simulink model "RRR_arm"  (R2017a)
settings: Solver=FixedStepAuto  StartTime=0.0  StopTime=15  FixedStep=0.1  RelTol=1e-3  EnableMultiTasking=on
settings Model: Creator=PaiChihYun  LastModifiedBy=tonypai
settings OptimizationCC: LifeSpan=inf
settings DebuggingCC: SFUnexpectedBacktrackingDiag=warning  SFNoUnconditionalDefaultTransitionDiag=warning  SFExecutionAtInitializationDiag=none
settings GRTTargetCC: TargetLangStandard=C89/C90 (ANSI)  GeneratePreprocessorConditionals=Disable all
settings ConfigComp: CovMetricSettings=dw  CovHtmlReporting=on  CovSaveCumulativeToWorkspaceVar=on  CovSaveSingleToWorkspaceVar=on  CovExternalEMLEnable=off

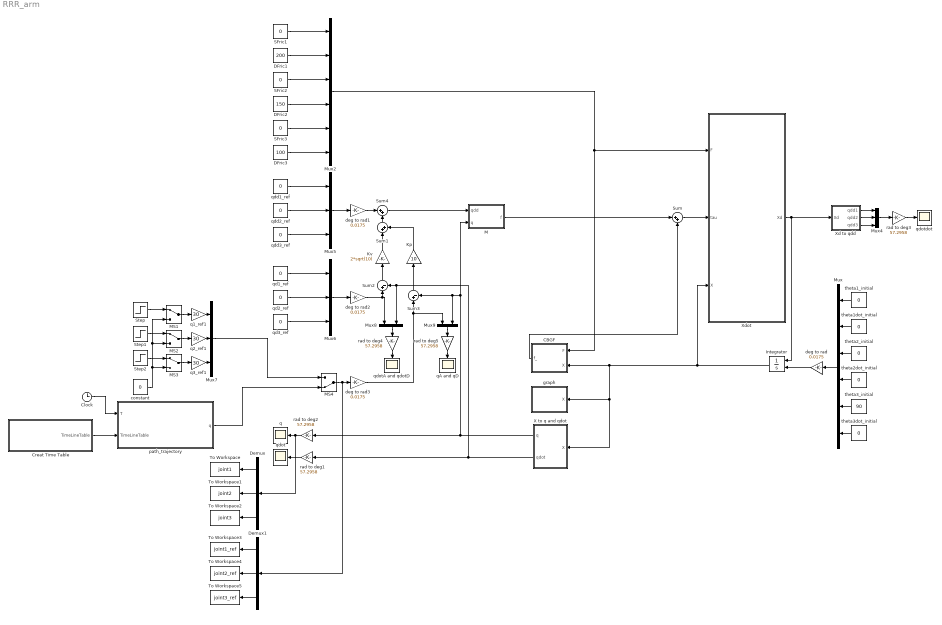
== system RRR_arm ==
  CBGF : MATLAB Function  TreatAsAtomicUnit=on
  Clock : Clock
  Creat Time Table : MATLAB Function  TreatAsAtomicUnit=on
  DFric1 : Constant  Value=200
  DFric2 : Constant  Value=150
  DFric3 : Constant  Value=100
  Demux : Demux  Outputs=3
  Demux1 : Demux  Outputs=3
  Integrator : Integrator  InitialConditionSource=external
  Kp : Gain  Gain=10
  Kv : Gain  Gain=2*sqrt(10)
  M : MATLAB Function  TreatAsAtomicUnit=on
  MS1 : ManualSwitch
  MS2 : ManualSwitch
  MS3 : ManualSwitch
  MS4 : ManualSwitch  CurrentSetting=0
  Mux : Mux  Inputs=6
  Mux2 : Mux  Inputs=6
  Mux{4..7} (4 alike) : Mux  Inputs=3
  Mux8 : Mux  Inputs=2
  Mux9 : Mux  Inputs=2
  SFric1 : Constant  Value=0
  SFric2 : Constant  Value=0
  SFric3 : Constant  Value=0
  Step : Step  Time=0  SampleTime=0
  Step1 : Step  Time=0  SampleTime=0
  Step2 : Step  Time=0  SampleTime=0
  Sum : Sum  Inputs=|++
  Sum1 : Sum  Inputs=|++
  Sum2 : Sum  Inputs=|+-
  Sum3 : Sum  Inputs=|+-
  Sum4 : Sum  Inputs=|++
  To Workspace : ToWorkspace  VariableName=joint1  SaveFormat=Timeseries  SampleTime=-1
  To Workspace1 : ToWorkspace  VariableName=joint2  SaveFormat=Timeseries  SampleTime=-1
  To Workspace2 : ToWorkspace  VariableName=joint3  SaveFormat=Timeseries  SampleTime=-1
  To Workspace3 : ToWorkspace  VariableName=joint1_ref  SaveFormat=Timeseries  SampleTime=-1
  To Workspace4 : ToWorkspace  VariableName=joint2_ref  SaveFormat=Timeseries  SampleTime=-1
  To Workspace5 : ToWorkspace  VariableName=joint3_ref  SaveFormat=Timeseries  SampleTime=-1
  X to q and qdot : MATLAB Function  TreatAsAtomicUnit=on
  Xd to qdd : MATLAB Function  TreatAsAtomicUnit=on
  Xdot : MATLAB Function  TreatAsAtomicUnit=on
  constant : Constant  Value=0
  deg to rad{,1..3} (4 alike) : Gain  Gain=0.0175
  graph : MATLAB Function  TreatAsAtomicUnit=on
  path_trajectory : MATLAB Function  TreatAsAtomicUnit=on
  q : Scope
  q1_ref1 : Gain  Gain=30
  q2_ref1 : Gain  Gain=30
  q3_ref1 : Gain  Gain=30
  qA and qD : Scope
  qd1_ref : Constant  Value=0
  qd2_ref : Constant  Value=0
  qd3_ref : Constant  Value=0
  qdd1_ref : Constant  Value=0
  qdd2_ref : Constant  Value=0
  qdd3_ref : Constant  Value=0
  qdot : Scope
  qdotA and qdotD : Scope
  qdotdot : Scope
  rad to deg{1..5} (5 alike) : Gain  Gain=57.2958
  theta1_initial : Constant  Value=0
  theta1dot_initial : Constant  Value=0
  theta2_initial : Constant  Value=0
  theta2dot_initial : Constant  Value=0
  theta3_initial : Constant  Value=90
  theta3dot_initial : Constant  Value=0
  wires:
  SFric2/1 -> Mux2/3
  DFric1/1 -> Mux2/2
  SFric1/1 -> Mux2/1
  Mux2/1 -> CBGF/1(F), Xdot/1(F)
  Xdot/1(Xd) -> Xd to qdd/1(Xd), Integrator/1
  theta3dot_initial/1 -> Mux/6
  theta3_initial/1 -> Mux/5
  theta2dot_initial/1 -> Mux/4
  theta2_initial/1 -> Mux/3
  theta1dot_initial/1 -> Mux/2
  theta1_initial/1 -> Mux/1
  Mux/1 -> deg to rad/1
  deg to rad/1 -> Integrator/2
  DFric3/1 -> Mux2/6
  SFric3/1 -> Mux2/5
  DFric2/1 -> Mux2/4
  X to q and qdot/2(qdot) -> Mux8/2, Sum2/2, rad to deg1/1
  rad to deg1/1 -> qdot/1
  Mux4/1 -> rad to deg3/1
  rad to deg3/1 -> qdotdot/1
  Xd to qdd/1(qdd1) -> Mux4/1
  Xd to qdd/2(qdd2) -> Mux4/2
  Xd to qdd/3(qdd3) -> Mux4/3
  Integrator/1 -> Xdot/3(X), X to q and qdot/1(X), graph/1(X), CBGF/2(X)
  CBGF/1(f_) -> Sum/2
  Kv/1 -> Sum1/1
  Kp/1 -> Sum1/2
  Sum3/1 -> Kp/1
  Sum2/1 -> Kv/1
  qd3_ref/1 -> Mux6/3
  qd2_ref/1 -> Mux6/2
  qd1_ref/1 -> Mux6/1
  q1_ref1/1 -> Mux7/1
  q2_ref1/1 -> Mux7/2
  q3_ref1/1 -> Mux7/3
  qdd1_ref/1 -> Mux5/1
  qdd2_ref/1 -> Mux5/2
  qdd3_ref/1 -> Mux5/3
  rad to deg2/1 -> Demux/1, q/1
  X to q and qdot/1(q) -> Mux9/2, Sum3/2, M/2(q), rad to deg2/1
  Sum4/1 -> M/1(qdd)
  Sum1/1 -> Sum4/2
  Mux5/1 -> deg to rad1/1
  Mux6/1 -> deg to rad2/1
  deg to rad1/1 -> Sum4/1
  deg to rad2/1 -> Mux8/1, Sum2/1
  deg to rad3/1 -> Mux9/1, Sum3/1
  Mux8/1 -> rad to deg4/1
  rad to deg4/1 -> qdotA and qdotD/1
  Mux9/1 -> rad to deg5/1
  rad to deg5/1 -> qA and qD/1
  Sum/1 -> Xdot/2(tau)
  M/1(f) -> Sum/1
  MS1/1 -> q1_ref1/1
  MS2/1 -> q2_ref1/1
  MS3/1 -> q3_ref1/1
  Step/1 -> MS1/1
  Step1/1 -> MS2/1
  Step2/1 -> MS3/1
  constant/1 -> MS1/2, MS2/2, MS3/2
  Demux/1 -> To Workspace/1
  Demux/2 -> To Workspace1/1
  Demux/3 -> To Workspace2/1
  Demux1/2 -> To Workspace4/1
  Demux1/3 -> To Workspace5/1
  Demux1/1 -> To Workspace3/1
  Creat Time Table/1(TimeLineTable) -> path_trajectory/2(TimeLineTable)
  Clock/1 -> path_trajectory/1(T)
  MS4/1 -> Demux1/1, deg to rad3/1
  Mux7/1 -> MS4/1
  path_trajectory/1(q) -> MS4/2

== matlab function RRR_arm/graph ==
  data: X input
function graph(X)
L1=4;
L2=3;
L3=2;
P0=[0;0;0;1];
q1=X(1);
q2=X(3);
q3=X(5);
c1=cos(q1);
c3=cos(q3);
s1=sin(q1);
s3=sin(q3);
c12=cos(q1+q2);
s12=sin(q1+q2);
joint1 = [P0(1);P0(2)];
joint2 = [L1*c1;L1*s1];
joint3 = [L2*(c12) + L1*c1;L2*(s12) + L1*s1];
joint4 = [L2*(c12) + L1*c1 + L3*(c3*(c12) - s3*(s12));L2*(s12) + L1*s1 + L3*(c3*(s12) + s3*(c12))];
hold off


plot([joint2(1);joint1(1)],[joint2(2);joint1(2)],'r','LineWidth',2);hold on
plot([joint3(1);joint2(1)],[joint3(2);joint2(2)],'g','LineWidth',2);hold on
plot([joint4(1);joint3(1)],[joint4(2);joint3(2)],'b','LineWidth',2);hold on
plot(joint1(1),joint1(2),'ko',joint2(1),joint2(2),'ko',joint3(1),joint3(2),'ko',joint4(1),joint4(2),'ko');hold on
title('RRR Robotic Arm Position'), xlabel('X'), ylabel('Y');grid on
axis_value = 10;
axis([-axis_value, axis_value, -axis_value, axis_value]);
end

== matlab function RRR_arm/Xdot ==
  data: F input; tau input; X input; Xd output
function Xd  = Xdot(F,tau,X)
g=9.81;
q1=X(1);
q1dot=X(2);
q2=X(3);
q2dot=X(4);
q3=X(5);
q3dot=X(6);
tau1=tau(1);
tau2=tau(2);
tau3=tau(3);

SFric1=F(1);
DFric1=F(2);
SFric2=F(3);
DFric2=F(4);
SFric3=F(5);
DFric3=F(6);
f1=SFric1*sign(q1dot) + DFric1*q1dot;
f2=SFric2*sign(q2dot) + DFric2*q2dot;
f3=SFric3*sign(q3dot) + DFric3*q3dot;
F=[f1;f2;f3];
%% -----------------------------------------------------------------%%
% c1=cos(q1);
% c2=cos(q2);
% c3=cos(q3);
% s2=sin(q2);
% s3=sin(q3);
% c12=cos(q1+q2);
% c23=cos(q2+q3);
% s23=sin(q2+q3);
% c123=cos(q1+q2+q3);

M=zeros(3,3);
M(1,1)=80*cos(q2+q3)+420*cos(q2)+60*cos(q3)+12291/20;
M(1,2)=40*cos(q2+q3)+210*cos(q2)+60*cos(q3)+2681/20;
M(1,3)=40*cos(q2+q3)+30*cos(q3)+101/10;
M(2,1)=40*cos(q2+q3)+210*cos(q2)+60*cos(q3)+2681/20;
M(2,2)=60*cos(q3)+2681*20;
M(2,3)=30*cos(q3)+101/10;
M(3,1)=40*cos(q2+q3)+30*cos(q3)+101/10;
M(3,2)=30*cos(q3)+101/10;
M(3,3)=101/10;

C=zeros(3,3);
C(1,2)=-40*sin(q2+q3)-210*sin(q2);
C(1,3)=-40*sin(q2+q3)-30*sin(q3);
C(2,1)=40*sin(q2+q3)+210*sin(q2);
C(2,3)=-30*sin(q3);
C(3,1)=40*sin(q2+q3)+30*sin(q3);
C(3,2)=30*sin(q3);

B=zeros(3,3);
B(1,1)=-80*sin(q2+q3)-420*sin(q2);
B(1,2)=-80*sin(q2+q3)-60*sin(q3);
B(1,3)=-80*sin(q2+q3)-60*sin(q3);
B(2,2)=-60*sin(q3);
B(2,3)=-60*sin(q3);
B(3,1)=60*sin(q3);

G=zeros(3,1);
G(1)=15*g*(3*cos(q1+q2)/2+4*cos(q1)) + 10*g*(cos(q1+q2+q3) + 3*cos(q1+q2) + 4*cos(q1)) + 40*g*cos(q1);
G(2)=10*g*(cos(q1+q2+q3) + 3*cos(q1+q2)) + (45*g*cos(q1+q2))/2;
G(3)=10*g*cos(q1+q2+q3);

qdd=M\([tau1;tau2;tau3] - C*[q1dot^2;q2dot^2;q3dot^2] - B*[q1dot*q2dot;q1dot*q3dot;q2dot*q3dot] - G - F );

Xd=zeros(6,1);
Xd(1)=q1dot;
Xd(2)=qdd(1);
Xd(3)=q2dot;
Xd(4)=qdd(2);
Xd(5)=q3dot;
Xd(6)=qdd(3);
end

== matlab function RRR_arm/X to q and qdot ==
  data: q output; qdot output; X input
function [q,qdot] =X_to_q(X)
q=[X(1);X(3);X(5)];
qdot=[X(2);X(4);X(6)];
end

== matlab function RRR_arm/Xd to qdd ==
  data: qdd1 output; qdd2 output; Xd input; qdd3 output
function [qdd1,qdd2,qdd3] =Xd_to_qd(Xd)
qdd1=Xd(2);
qdd2=Xd(4);
qdd3=Xd(6);
end

== matlab function RRR_arm/M ==
  data: qdd input; q input; f output
function f = M(qdd,q)
% q1=q(1);
q2=q(2);
q3=q(3);
M=zeros(3,3);
M(1,1)=80*cos(q2+q3)+420*cos(q2)+60*cos(q3)+12291/20;
M(1,2)=40*cos(q2+q3)+210*cos(q2)+60*cos(q3)+2681/20;
M(1,3)=40*cos(q2+q3)+30*cos(q3)+101/10;
M(2,1)=40*cos(q2+q3)+210*cos(q2)+60*cos(q3)+2681/20;
M(2,2)=60*cos(q3)+2681*20;
M(2,3)=30*cos(q3)+101/10;
M(3,1)=40*cos(q2+q3)+30*cos(q3)+101/10;
M(3,2)=30*cos(q3)+101/10;
M(3,3)=101/10;
f=M*[qdd(1);qdd(2);qdd(3)];
end

== matlab function RRR_arm/CBGF ==
  data: F input; f_ output; X input
function f_ = CBGF(F,X)
g=9.81;
q1=X(1);
q1dot=X(2);
q2=X(3);
q2dot=X(4);
q3=X(5);
q3dot=X(6);
SFric1=F(1);
DFric1=F(2);
SFric2=F(3);
DFric2=F(4);
SFric3=F(5);
DFric3=F(6);
f1=SFric1*sign(q1dot) + DFric1*q1dot;
f2=SFric2*sign(q2dot) + DFric2*q2dot;
f3=SFric3*sign(q3dot) + DFric3*q3dot;
F=[f1;f2;f3];

C=zeros(3,3);
C(1,2)=-40*sin(q2+q3)-210*sin(q2);
C(1,3)=-40*sin(q2+q3)-30*sin(q3);
C(2,1)=40*sin(q2+q3)+210*sin(q2);
C(2,3)=-30*sin(q3);
C(3,1)=40*sin(q2+q3)+30*sin(q3);
C(3,2)=30*sin(q3);

B=zeros(3,3);
B(1,1)=-80*sin(q2+q3)-420*sin(q2);
B(1,2)=-80*sin(q2+q3)-60*sin(q3);
B(1,3)=-80*sin(q2+q3)-60*sin(q3);
B(2,2)=-60*sin(q3);
B(2,3)=-60*sin(q3);
B(3,1)=60*sin(q3);

G=zeros(3,1);
G(1)=15*g*(3*cos(q1+q2)/2+4*cos(q1)) + 10*g*(cos(q1+q2+q3) + 3*cos(q1+q2) + 4*cos(q1)) + 40*g*cos(q1);
G(2)=10*g*(cos(q1+q2+q3) + 3*cos(q1+q2)) + (45*g*cos(q1+q2))/2;
G(3)=10*g*cos(q1+q2+q3);

f_ = C*[q1dot^2;q2dot^2;q3dot^2] + B*[q1dot*q2dot;q1dot*q3dot;q2dot*q3dot] + G + F;
end

== matlab function RRR_arm/path_trajectory ==
  data: T input; q output; TimeLineTable input
function q   = path_trajectory(T,TimeLineTable)
[~, index] = min(abs(T-TimeLineTable(:,1)));
q = TimeLineTable(index,2:4)';
end

== matlab function RRR_arm/Creat Time Table ==
  data: TimeLineTable output
function TimeLineTable =CreatTimeTable()
TimeLineTable_initial=[0,0,0,90;2,30,-10,70;4,45,130,-85;6,150,10,70;8,180,0,-90];
T=TimeLineTable_initial(:,1);
joint1=spline(T,[0, TimeLineTable_initial(:,2)', 0]);
joint2=spline(T,[0, TimeLineTable_initial(:,3)', 0]);
joint3=spline(T,[0, TimeLineTable_initial(:,4)', 0]);
Ts=min(T):.01:max(T);
TimeLineTable=[Ts',ppval(joint1,Ts)',ppval(joint2,Ts)',ppval(joint3,Ts)'];
end
